simulink model "sim_levitador"  (R2019b)
settings: Solver=VariableStepAuto  StartTime=0.0  StopTime=10.0  RelTol=1e-3
values from neighbouring files (symbols this model uses):
  a = 0.04939    [dev_levitador.m]    (also in sim_levitador.m = 1)
  g = 9.81    [dev_levitador.m]    (also in sim_levitador.m)
  Ls = 0.014    [dev_levitador.m]    (also in sim_levitador.m = 1)
  m = 0.025    [dev_levitador.m]    (also in sim_levitador.m = 1)
  Ts = 0.001    [sim_levitador.m]
settings Model: Creator=tronc  LastModifiedBy=tronc
settings DataIOCC: SaveFormat=Array

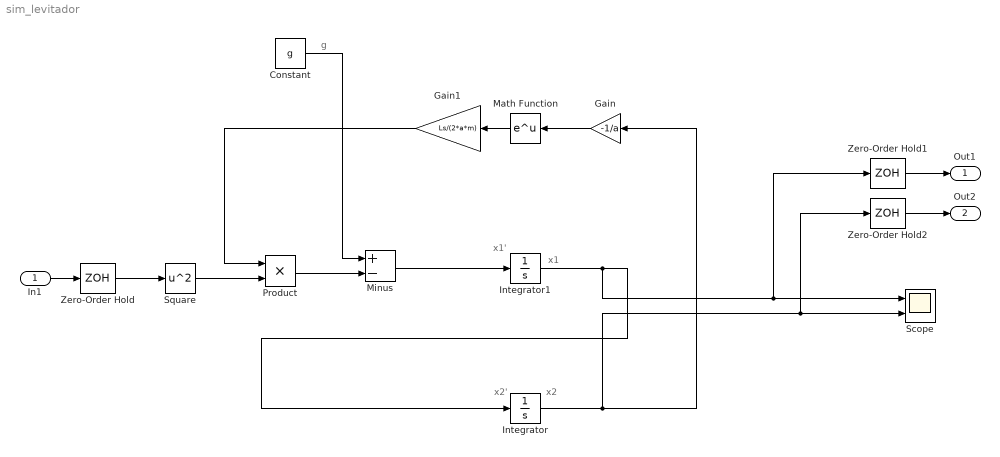
== system sim_levitador ==
  note: x2'
  note: x1
  note: x2
  note: x1'
  note: g
  In1 : Inport
  Constant : Constant  Value=g
  Gain : Gain  Gain=-1/a
  Gain1 : Gain  Gain=Ls/(2*a*m)
  Integrator : Integrator
  Integrator1 : Integrator
  Math Function : Math  SignedPower=off  SaturateOnIntegerOverflow=on
  Minus : Sum  Inputs=+-
  Product : Product
  Scope : Scope  NumInputPorts=2
  Square : Math  Operator=square  SignedPower=off  SaturateOnIntegerOverflow=on
  Zero-Order Hold : ZeroOrderHold  SampleTime=Ts
  Zero-Order Hold1 : ZeroOrderHold  SampleTime=Ts
  Zero-Order Hold2 : ZeroOrderHold  SampleTime=Ts
  Out1 : Outport
  Out2 : Outport  Port=2
  wires:
  Integrator1/1 -> Zero-Order Hold1/1, Scope/1, Integrator/1
  Minus/1 -> Integrator1/1
  Constant/1 -> Minus/1
  Gain/1 -> Math Function/1
  Math Function/1 -> Gain1/1
  Gain1/1 -> Product/1
  Square/1 -> Product/2
  Zero-Order Hold/1 -> Square/1
  Product/1 -> Minus/2
  Integrator/1 -> Zero-Order Hold2/1, Scope/2, Gain/1
  In1/1 -> Zero-Order Hold/1
  Zero-Order Hold1/1 -> Out1/1
  Zero-Order Hold2/1 -> Out2/1
